simulink model "PassStCshnFldHolderChk"  (R2018b)
settings: Solver=FixedStepDiscrete  StartTime=0.0  StopTime=10.0  RelTol=1e-3
settings Model: ModifiedHistory=2024.6.26 V3.0.0 557模式流程  Creator=sn2xws  LastModifiedBy=sn2xws
settings DataIOCC: SaveFormat=StructureWithTime
settings OptimizationCC: DefaultParameterBehavior=Inlined  EnhancedBackFolding=on  PassReuseOutputArgsAs=Individual arguments  ZeroExternalMemoryAtStartup=off  ZeroInternalMemoryAtStartup=off  OptimizeBlockOrder=speed  DifferentSizesBufferReuse=on  OptimizationCustomize=off
settings DebuggingCC: ParameterTunabilityLossMsg=error
settings SFSimCC: MATLABDynamicMemAlloc=off
settings RTWCC: SystemTargetFile=autosar.tlc  GenCodeOnly=on  TemplateMakefile=ert_default_tmf  Description=AUTOSAR  GenerateReport=on  IncludeHyperlinkInReport=on  LaunchReport=on  GenerateTraceInfo=on  GenerateTraceReport=on  GenerateTraceReportSl=on  GenerateTraceReportSf=on  GenerateTraceReportEml=on
settings CodeAppCC: ForceParamTrailComments=on  IgnoreCustomStorageClasses=off  OperatorAnnotations=on  SimulinkDataObjDesc=on  SFDataObjDesc=on  InsertBlockDesc=on
settings STFCustomTargetCC: TargetLangStandard=C99 (ISO)  MultiwordLength=256  ParMdlRefBuildCompliant=on  CompOptLevelCompliant=on  IncludeMdlTerminateFcn=off  CombineOutputUpdateFcns=on  SuppressErrorStatus=on  ERTCustomFileBanners=on  SupportNonFinite=off  SupportComplex=off  SupportContinuousTime=off  SupportNonInlinedSFcns=off  RemoveResetFunc=on  MATLABClassNameForMDSCustomization=Simulink.SoftwareTarget.ERTCustomization  AutosarCompliant=on  UseToolchainInfoCompliant=on  LookupTableObjectStructAxisOrder=2,1,3,4,...  LUTObjectStructOrderEvenSpacing=Size,Table,Breakpoints  SystemTargetFile=autosar.tlc
settings ERTTargetCC: TargetLangStandard=C99 (ISO)  ConcurrentExecutionCompliant=off  IncludeMdlTerminateFcn=off  SuppressErrorStatus=on  SupportNonFinite=off  SupportComplex=off  ModelStepFunctionPrototypeControlCompliant=off  CPPClassGenCompliant=off  AutosarCompliant=on  LookupTableObjectStructAxisOrder=2,1,3,4,...  LUTObjectStructOrderEvenSpacing=Size,Table,Breakpoints  InlinedParameterPlacement=NonHierarchical  ERTCustomFileTemplate=example_file_process.tlc  ERTFilePackagingFormat=Compact

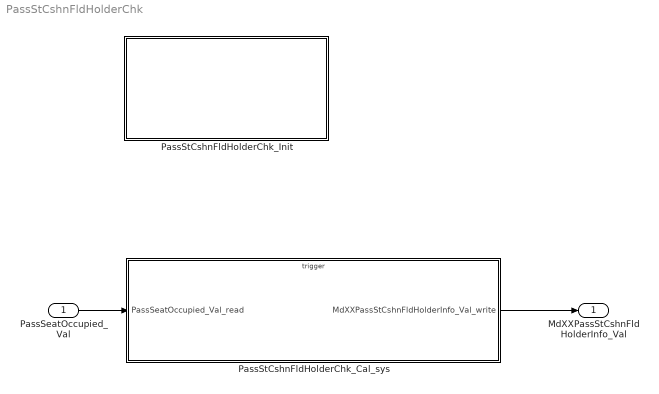
== system PassStCshnFldHolderChk ==
  PassSeatOccupied_Val : Inport  OutDataTypeStr=boolean  PortDimensions=1
  PassStCshnFldHolderChk_Cal_sys : Subsystem
  PassStCshnFldHolderChk_Init : Subsystem
  MdXXPassStCshnFldHolderInfo_Val : Outport  OutDataTypeStr=uint32  PortDimensions=1
  wires:
  PassSeatOccupied_Val/1 -> PassStCshnFldHolderChk_Cal_sys/1(PassSeatOccupied_Val_read)
  PassStCshnFldHolderChk_Cal_sys/1(MdXXPassStCshnFldHolderInfo_Val_write) -> MdXXPassStCshnFldHolderInfo_Val/1

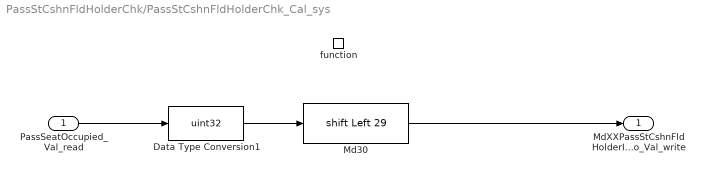
== system PassStCshnFldHolderChk/PassStCshnFldHolderChk_Cal_sys ==
  PassSeatOccupied_Val_read : Inport
  function : TriggerPort  TriggerType=function-call  IsSimulinkFunction=on  FunctionName=PassStCshnFldHolderChk_Cal  VariantControl=(inherit)
  Data Type Conversion1 : DataTypeConversion  OutDataTypeStr=uint32
  Md30 : ArithShift  BitShiftNumber=29  BitShiftDirection=Left
  MdXXPassStCshnFldHolderInfo_Val_write : Outport
      settings: EnsureOutportIsVirtual=on
  wires:
  Md30/1 -> MdXXPassStCshnFldHolderInfo_Val_write/1
  PassSeatOccupied_Val_read/1 -> Data Type Conversion1/1
  Data Type Conversion1/1 -> Md30/1

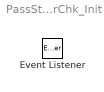
== system PassStCshnFldHolderChk/PassStCshnFldHolderChk_Init ==
  Event Listener : EventListener  EventName=reset
